simulink model "q2"  (R2020b)
settings: Solver=VariableStepAuto  StartTime=0.0  StopTime=100.0  MaxStep=0.001  RelTol=1e-3
values from neighbouring files (symbols this model uses):
  b = 7    [p1init.m]
  k1 = 0.5    [p1init.m]
  k2 = 0.6    [p1init.m]
  m1 = 200    [p1init.m]
  m2 = 5    [p1init.m]
settings Model: Creator=Vrunda M Balgi  LastModifiedBy=Vrunda M Balgi
settings DataIOCC: LoadExternalInput=on

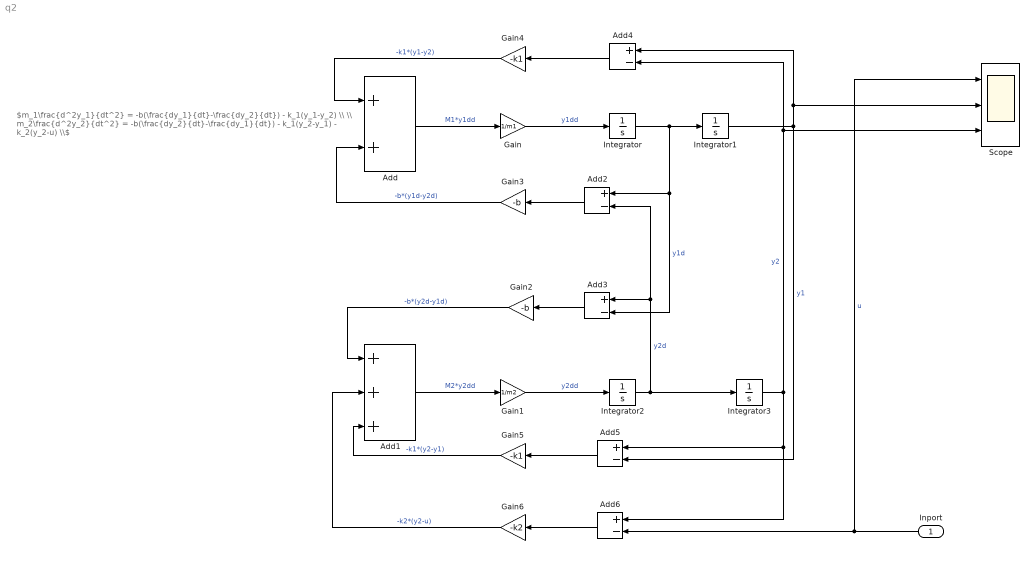
== system q2 ==
  note: $m_1\frac{d^2y_1}{dt^2} = -b(\frac{dy_1}{dt}-\frac{dy_2}{dt}) - k_1(y_1-y_2) \\ \\ m_2\frac{d^2y_2}{dt^2} = -b(\frac{dy_2}{dt}-\frac{dy_1}{dt}) - k_1(y_2-y_1) - k_2(y_2-u) \\$
  Inport : Inport
  Add : Sum
  Add1 : Sum  Inputs=+++
  Add{2..6} (5 alike) : Sum  Inputs=+-
  Gain : Gain  Gain=1/m1
  Gain1 : Gain  Gain=1/m2
  Gain2 : Gain  Gain=-b
  Gain3 : Gain  Gain=-b
  Gain4 : Gain  Gain=-k1
  Gain5 : Gain  Gain=-k1
  Gain6 : Gain  Gain=-k2
  Integrator{,1..3} (4 alike) : Integrator
  Scope : Scope  NumInputPorts=3
  wires:
  Add/1 -> Gain/1  "M1*y1dd"
  Gain/1 -> Integrator/1  "y1dd"
  Integrator/1 -> Add3/2, Add2/1, Integrator1/1  "y1d"
  Integrator1/1 -> Add4/1, Scope/2, Add5/2  "y1"
  Add1/1 -> Gain1/1  "M2*y2dd"
  Gain1/1 -> Integrator2/1  "y2dd"
  Integrator2/1 -> Integrator3/1, Add3/1, Add2/2  "y2d"
  Add2/1 -> Gain3/1
  Add3/1 -> Gain2/1
  Gain3/1 -> Add/2  "-b*(y1d-y2d)"
  Gain2/1 -> Add1/1  "-b*(y2d-y1d)"
  Integrator3/1 -> Add4/2, Scope/3, Add5/1, Add6/1  "y2"
  Add4/1 -> Gain4/1
  Gain4/1 -> Add/1  "-k1*(y1-y2)"
  Add5/1 -> Gain5/1
  Gain5/1 -> Add1/3  "-k1*(y2-y1)"
  Add6/1 -> Gain6/1
  Inport/1 -> Scope/1, Add6/2  "u"
  Gain6/1 -> Add1/2  "-k2*(y2-u)"
